simulink model "exsim6_ss_observer_model"  (R2018b)
settings: Solver=VariableStepAuto  StartTime=0.0  StopTime=10.0  FixedStep=Ts  RelTol=1e-3
values from neighbouring files (symbols this model uses):
  A = [0 1; 0.16 -1]    [exsim6.m]
  B = [0 1]'    [exsim6.m]
  C = [1 0]    [exsim6.m]
  N = 1    [exsim6.m]
  nF = double(linsolve(m,v)')    [exsim6.m]
  nL = double(linsolve(m,v))    [exsim6.m]
settings Model: Creator=rafael  LastModifiedBy=rafael

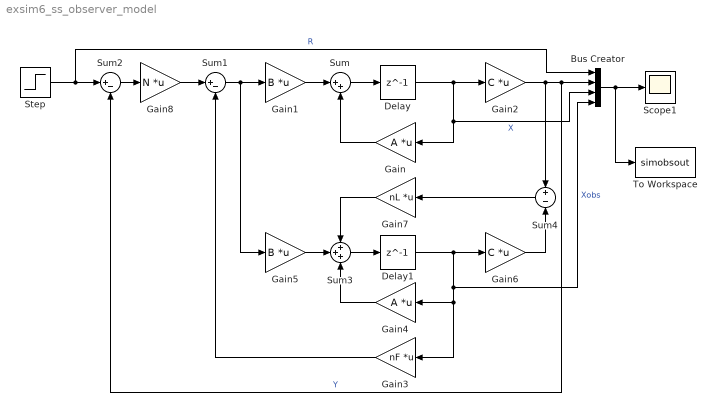
== system exsim6_ss_observer_model ==
  Bus Creator : BusCreator  Inputs=4
  Delay : Delay  DelayLength=1
  Delay1 : Delay  DelayLength=1
  Gain : Gain  Gain=A  Multiplication=Matrix(K*u)
  Gain1 : Gain  Gain=B  Multiplication=Matrix(K*u)
  Gain2 : Gain  Gain=C  Multiplication=Matrix(K*u)
  Gain3 : Gain  Gain=nF  Multiplication=Matrix(K*u)
  Gain4 : Gain  Gain=A  Multiplication=Matrix(K*u)
  Gain5 : Gain  Gain=B  Multiplication=Matrix(K*u)
  Gain6 : Gain  Gain=C  Multiplication=Matrix(K*u)
  Gain7 : Gain  Gain=nL  Multiplication=Matrix(K*u)
  Gain8 : Gain  Gain=N  Multiplication=Matrix(K*u)
  Scope1 : Scope
  Step : Step  SampleTime=0
  Sum : Sum  Inputs=|++
  Sum1 : Sum  Inputs=|+-
  Sum2 : Sum  Inputs=|+-
  Sum3 : Sum  Inputs=+++
  Sum4 : Sum  Inputs=+|-
  To Workspace : ToWorkspace  VariableName=simobsout  SaveFormat=Timeseries  SampleTime=-1
  wires:
  Sum/1 -> Delay/1
  Gain/1 -> Sum/2
  Gain1/1 -> Sum/1
  Delay/1 -> Gain2/1, Bus Creator/3, Gain/1  "X"
  Gain2/1 -> Bus Creator/2, Sum2/2, Sum4/1  "Y"
  Sum3/1 -> Delay1/1
  Sum4/1 -> Gain7/1
  Gain6/1 -> Sum4/2
  Gain7/1 -> Sum3/1
  Gain5/1 -> Sum3/2
  Gain4/1 -> Sum3/3
  Gain3/1 -> Sum1/2
  Sum1/1 -> Gain5/1, Gain1/1
  Gain8/1 -> Sum1/1
  Sum2/1 -> Gain8/1
  Bus Creator/1 -> Scope1/1, To Workspace/1
  Step/1 -> Bus Creator/1, Sum2/1  "R"
  Delay1/1 -> Gain3/1, Gain4/1, Bus Creator/4, Gain6/1  "Xobs"
